simulink model "ex3sim"  (R2017a)
settings: Solver=ode45  StartTime=0.0  StopTime=15  MaxStep=1e-2  RelTol=1e-3  EnableMultiTasking=on
values from neighbouring files (symbols this model uses):
  K = 1    [ex3.m]
  Kp = f*alpha*[1 0; 0 -1]*[cos(phi) sin(phi); -sin(phi) cos(phi)]/z0    [ex3.m]
  q0 = [-pi/20 -pi/2]'    [ex3.m]
  x_c0 = -Kp*p_bc + O_c    [ex3.m]
libraries: roblocks x3, dspmtrx3 x2
settings Model: Creator=alexfneves  LastModifiedBy=rbp
settings DataIOCC: LimitDataPoints=on  SaveFormat=Array
settings OptimizationCC: LifeSpan=inf
settings DebuggingCC: SFUnexpectedBacktrackingDiag=warning  SFNoUnconditionalDefaultTransitionDiag=warning  SFExecutionAtInitializationDiag=none
settings HardwareCC: ProdBitPerPointer=32  ProdBitPerSizeT=32  ProdBitPerPtrDiffT=32  ProdLargestAtomicFloat=None  ProdIntDivRoundTo=Undefined  ProdEndianess=Unspecified  ProdWordSize=32  ProdHWDeviceType=32-bit Generic
settings ModelReferenceCC: PropagateSignalLabelsOutOfModel=off
settings GRTTargetCC: TargetLangStandard=C89/C90 (ANSI)  GeneratePreprocessorConditionals=Disable all
settings ConfigComp: CovMetricSettings=dw  CovHtmlReporting=on  CovSaveCumulativeToWorkspaceVar=on  CovSaveSingleToWorkspaceVar=on  CovExternalEMLEnable=off

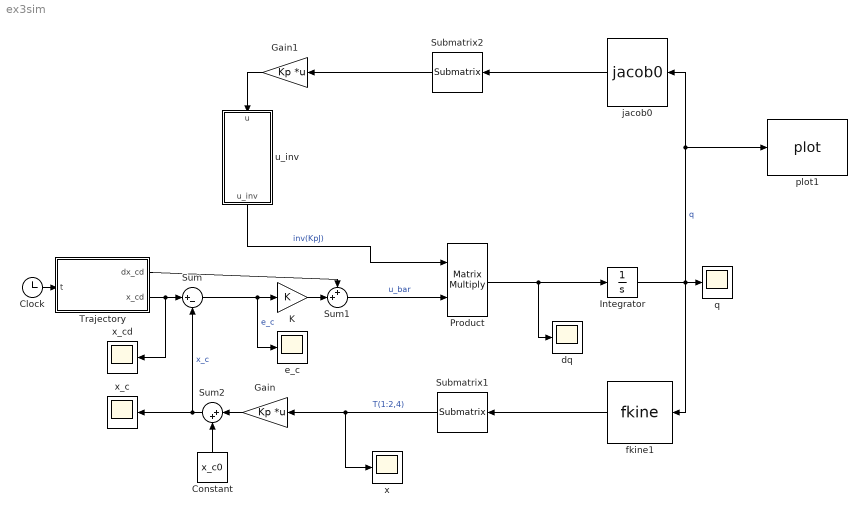
== system ex3sim ==
  Clock : Clock
  Constant : Constant  Value=x_c0
  Gain : Gain  Gain=Kp  Multiplication=Matrix(K*u)
  Gain1 : Gain  Gain=Kp  Multiplication=Matrix(K*u)
  Integrator : Integrator  InitialCondition=q0
  K : Gain  Gain=K
  Product : Product  Multiplication=Matrix(*)
  Submatrix1 : dspmtrx3/Submatrix  RowSpan=Range of rows  RowStartMode=First  RowStartIndex=1  RowEndMode=Index  RowEndIndex=2  ColSpan=One column  ColStartMode=Last  ColStartIndex=1  ColEndMode=Last  ColEndIndex=1
  Submatrix2 : dspmtrx3/Submatrix  RowSpan=Range of rows  RowStartMode=First  RowStartIndex=1  RowEndMode=Index  RowEndIndex=2  ColSpan=All columns  ColStartMode=First  ColStartIndex=1  ColEndMode=Index  ColEndIndex=2
  Sum : Sum  Inputs=|+-
  Sum1 : Sum  Inputs=++|
  Sum2 : Sum  Inputs=|++
  Trajectory : MATLAB Function  TreatAsAtomicUnit=on
  dq : Scope
  e_c : Scope
  fkine1 : roblocks/Arm/fkine  robot=planar
  "jacob0 " : roblocks/Arm/jacob0   robot=planar
  plot1 : roblocks/Arm/plot  robot=planar  fps=5  holdplot=on
  q : Scope
  u_inv : MATLAB Function  TreatAsAtomicUnit=on
  x : Scope
  x_c : Scope
  x_cd : Scope
  wires:
  Integrator/1 -> plot1/1, "jacob0 "/1, fkine1/1, q/1  "q"
  Sum/1 -> e_c/1, K/1  "e_c"
  Clock/1 -> Trajectory/1(t)
  fkine1/1 -> Submatrix1/1
  Trajectory/2(x_cd) -> x_cd/1, Sum/1
  K/1 -> Sum1/2
  Trajectory/1(dx_cd) -> Sum1/1
  Sum1/1 -> Product/2  "u_bar"
  Product/1 -> Integrator/1, dq/1
  Submatrix1/1 -> Gain/1, x/1  "T(1:2,4)"
  Sum2/1 -> Sum/2, x_c/1  "x_c"
  Gain/1 -> Sum2/1
  u_inv/1(u_inv) -> Product/1  "inv(KpJ)"
  Gain1/1 -> u_inv/1(u)
  "jacob0 "/1 -> Submatrix2/1
  Submatrix2/1 -> Gain1/1
  Constant/1 -> Sum2/2

== matlab function ex3sim/u_inv ==
  data: u input; u_inv output
function u_inv = fcn(u)
%#codegen

u_inv = inv(u);

== matlab function ex3sim/Trajectory ==
  data: dx_cd output; x_cd output; t input
function [dx_cd, x_cd] = trajectory(t)
%#codegen

    x_cd = x_cdFunc(t);
    dx_cd = dx_cdFunc(t);
end
